simulink model "um_simulation_experiment"  (Simulink 8.1)
settings: Solver=ode8  StartTime=0.0  StopTime=70  RelTol=1e-3
settings Model: Creator=petter  LastModifiedBy=petter
settings DataIOCC: SaveOutput=off  SaveTime=off
settings OptimizationCC: ExpressionDepthLimit=128
settings DebuggingCC: MultiTaskDSMMsg=warning  MultiTaskCondExecSysMsg=none  FcnCallInpInsideContextMsg=EnableAllAsError
settings RTWCC: IncludeERTFirstTime=on
settings GRTTargetCC: CombineOutputUpdateFcns=on  GRTInterface=off

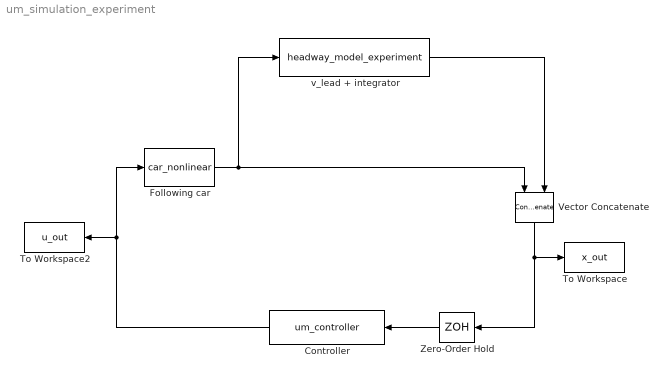
== system um_simulation_experiment ==
  Controller : M-S-Function  FunctionName=um_controller
  Following car : M-S-Function  FunctionName=car_nonlinear  Parameters=0
  To Workspace : ToWorkspace  VariableName=x_out  SampleTime=-1  SaveFormat=Structure With Time
  To Workspace2 : ToWorkspace  VariableName=u_out  SampleTime=-1  SaveFormat=Structure With Time
  Vector Concatenate : Concatenate
  Zero-Order Hold : ZeroOrderHold  SampleTime=0.01
  v_lead + integrator : M-S-Function  FunctionName=headway_model_experiment  Parameters=0
  wires:
  Controller/1 -> Following car/1, To Workspace2/1
  Zero-Order Hold/1 -> Controller/1
  Vector Concatenate/1 -> To Workspace/1, Zero-Order Hold/1
  Following car/1 -> v_lead + integrator/1, Vector Concatenate/1
  v_lead + integrator/1 -> Vector Concatenate/2
